simulink model "ljsvdp"  (Simulink 4.00)
settings: Solver=ode45  SolverMode=SingleTasking  StartTime=0.0  StopTime=500  RelTol=1e-3  AbsTol=1e-6
libraries: simulink3 x1
settings Model: LastModifiedBy=LJS  LimitDataPoints=off

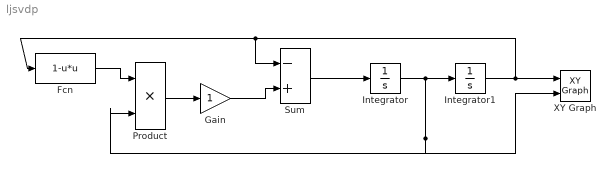
== system ljsvdp ==
  Fcn : Fcn  Expr=1-u*u
  Gain : Gain  Gain=1  Multiplication=Element-wise(K.*u)  SaturateOnIntegerOverflow=on
  Integrator : Integrator  ExternalReset=none  InitialConditionSource=internal  InitialCondition=0.1  LimitOutput=off  UpperSaturationLimit=inf  LowerSaturationLimit=-inf  ShowSaturationPort=off  ShowStatePort=off  AbsoluteTolerance=auto
  Integrator1 : Integrator  ExternalReset=none  InitialConditionSource=internal  InitialCondition=0  LimitOutput=off  UpperSaturationLimit=inf  LowerSaturationLimit=-inf  ShowSaturationPort=off  ShowStatePort=off  AbsoluteTolerance=auto
  Product : Product  Inputs=2  Multiplication=Element-wise(.*)  SaturateOnIntegerOverflow=on
  Sum : Sum  Inputs=-+  SaturateOnIntegerOverflow=on
  XY Graph : simulink3/Sinks/XY Graph  xmin=-5  xmax=5  ymin=-5  ymax=5  st=0.01
  wires:
  Sum/1 -> Integrator/1
  Gain/1 -> Sum/2
  Product/1 -> Gain/1
  Integrator1/1 -> XY Graph/1, Sum/1, Fcn/1
  Integrator/1 -> Integrator1/1, XY Graph/2, Product/2
  Fcn/1 -> Product/1
